simulink model "control_simulation_A"  (R2018a)
settings: Solver=ode8  StartTime=0.0  StopTime=sm_time  FixedStep=Ts  RelTol=1e-3
undefined symbols (not defined in the file): Gains, param, t_T, t_w, Tref, wref
libraries: cstblocks x1
settings Model: Creator=eduar  LastModifiedBy=eduar

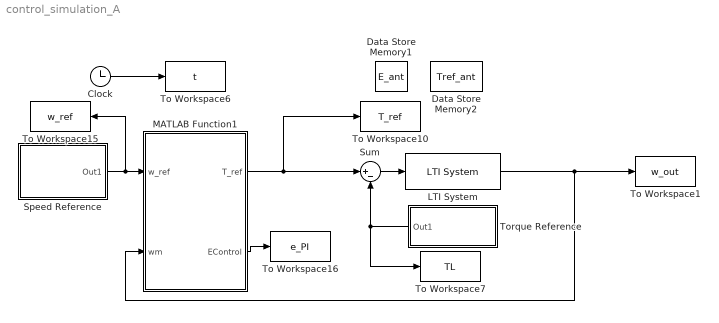
== system control_simulation_A ==
  Clock : Clock
  Data Store Memory1 : DataStoreMemory  DataStoreName=E_ant  InitialValue=1  ShowAdditionalParam=off  OutDataTypeStr=double
  Data Store Memory2 : DataStoreMemory  DataStoreName=Tref_ant  InitialValue=1  ShowAdditionalParam=off  OutDataTypeStr=double
  LTI System : cstblocks/LTI System  sys=RotorTF  IC=[]
  MATLAB Function1 : MATLAB Function  TreatAsAtomicUnit=on
  Speed Reference : Subsystem
  Sum : Sum  Inputs=|+-
  To Workspace1 : ToWorkspace  VariableName=w_out  SampleTime=-1
  To Workspace10 : ToWorkspace  VariableName=T_ref  SampleTime=-1
  To Workspace15 : ToWorkspace  VariableName=w_ref  SampleTime=-1
  To Workspace16 : ToWorkspace  VariableName=e_PI  SampleTime=-1
  To Workspace6 : ToWorkspace  VariableName=t  SampleTime=-1
  To Workspace7 : ToWorkspace  VariableName=TL  SampleTime=-1
  Torque Reference : Subsystem
  wires:
  Clock/1 -> To Workspace6/1
  Speed Reference/1(Out1) -> To Workspace15/1, MATLAB Function1/1(w_ref)
  MATLAB Function1/1(T_ref) -> Sum/1, To Workspace10/1
  MATLAB Function1/2(EControl) -> To Workspace16/1
  Sum/1 -> LTI System/1
  Torque Reference/1(Out1) -> To Workspace7/1, Sum/2
  LTI System/1 -> To Workspace1/1, MATLAB Function1/2(wm)

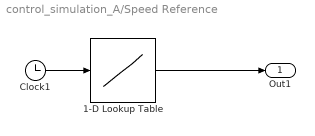
== system control_simulation_A/Speed Reference ==
  1-D Lookup Table : Lookup_n-D  NumberOfTableDimensions=1  BreakpointsForDimension1=t_w  Table=wref  InternalRulePriority=Speed  RndMeth=Simplest  InputSameDT=on
  Clock1 : Clock
  Out1 : Outport
  wires:
  Clock1/1 -> 1-D Lookup Table/1
  1-D Lookup Table/1 -> Out1/1

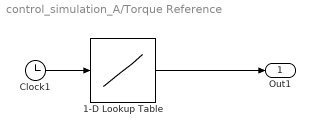
== system control_simulation_A/Torque Reference ==
  1-D Lookup Table : Lookup_n-D  NumberOfTableDimensions=1  BreakpointsForDimension1=t_T  Table=Tref  InterpMethod=Nearest  InternalRulePriority=Speed  RndMeth=Simplest  InputSameDT=on
  Clock1 : Clock
  Out1 : Outport
  wires:
  Clock1/1 -> 1-D Lookup Table/1
  1-D Lookup Table/1 -> Out1/1

== matlab function control_simulation_A/MATLAB Function1 ==
  settings: updateMethod=DISCRETE  sampleTime=Ts
  data: T_ref output; w_ref input; EControl output; wm input; Tref_ant data_store_memory; E_ant data_store_memory; param parameter; Gains parameter
function [T_ref, EControl] = fcn(w_ref, wm, param, Gains)
    global Tref_ant E_ant
    T_nom = param.T_nom;
    EControl = w_ref - wm;
    T_ref = Gains(1)*EControl + Gains(2)*E_ant + Gains(3)*Tref_ant;
    Tref_ant = T_ref; E_ant = EControl;
    
    if abs(T_ref) > abs(T_nom*2)
        if T_ref > 0
            T_ref = T_nom*2;
        elseif T_ref < 0
            T_ref = -1*T_nom*2;
        end
    end
